simulink model "aracer"  (R2024b)
settings: Solver=FixedStepAuto  StartTime=0.0  StopTime=10.0  RelTol=1e-3
libraries: robotlib x4, simulink x2
settings Model: Creator=mrudi  LastModifiedBy=mrudi
settings OptimizationCC: DefaultParameterBehavior=Inlined  EnhancedBackFolding=on  PassReuseOutputArgsAs=Individual arguments  ZeroExternalMemoryAtStartup=off  ZeroInternalMemoryAtStartup=off  MaxStackSize=64  OptimizeBlockOrder=speed  DifferentSizesBufferReuse=on  OptimizationCustomize=off  EfficientTunableParamExpr=on
settings DebuggingCC: ParameterTunabilityLossMsg=error
settings HardwareCC: ProdBitPerPointer=32  ProdBitPerSizeT=32  ProdBitPerPtrDiffT=32  ProdLargestAtomicFloat=None  ProdIntDivRoundTo=Undefined  ProdEndianess=Unspecified  ProdWordSize=32  ProdHWDeviceType=Generic->Unspecified (assume 32-bit Generic)  UseEmbeddedCoderFeatures=off
settings SFSimCC: MATLABDynamicMemAlloc=off
settings RTWCC: Description=Embedded Coder  SystemTargetFile=ert.tlc  HardwareBoard=Robot Operating System (ROS)  TLCOptions="-aInlineSetEventsForThisBaseRateFcn=TLC_FALSE -aSuppressMultiTaskScheduler=TLC_FALSE  -aRateBasedStepFcn=0"  GenCodeOnly=on  TemplateMakefile=ert_default_tmf  Toolchain=Catkin  TargetLang=C++
settings CodeAppCC: ForceParamTrailComments=on  IgnoreCustomStorageClasses=off  OperatorAnnotations=on  SimulinkDataObjDesc=on  SFDataObjDesc=on  InsertBlockDesc=on
settings ERTTargetCC: SupportNonInlinedSFcns=on

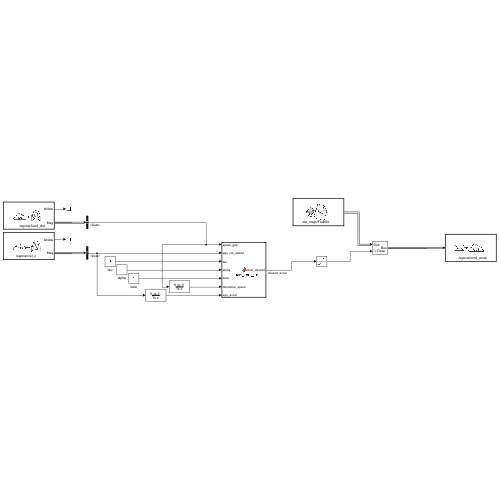
[thumbnail: Simulink's stored preview of the top-level diagram]
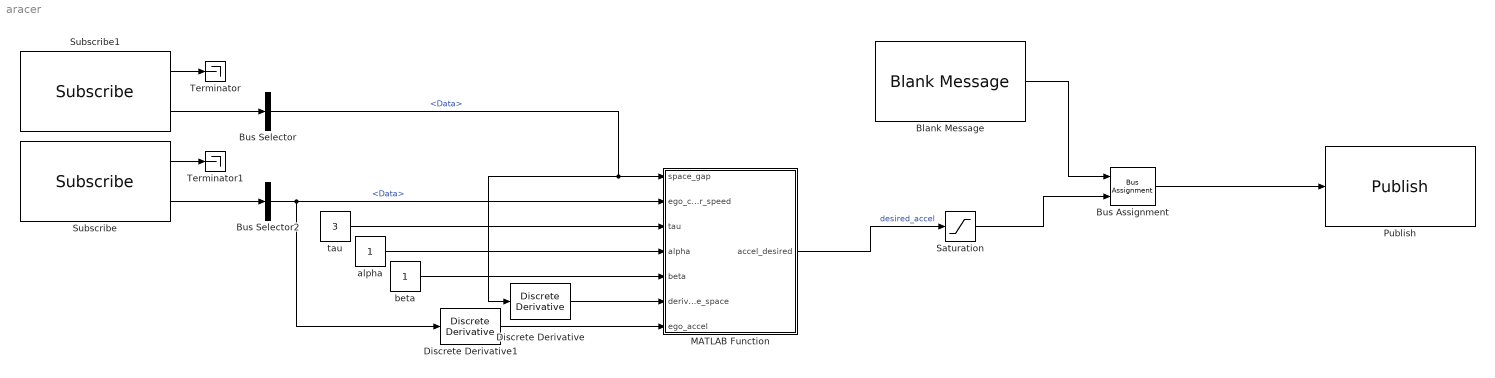
== system aracer ==
  Blank Message : robotlib/Blank Message  messageClass=Message  entityType=std_msgs/Float64  messageType=std_msgs/Float64  SampleTime=inf  legacyBusStruct=off
  Bus Assignment : BusAssignment  AssignedSignals=Data
  Bus Selector : BusSelector  OutputSignals=Data
  Bus Selector2 : BusSelector  OutputSignals=Data
  Discrete Derivative : simulink/Discrete/Discrete Derivative  gainval=1.0  ICPrevScaledInput=0.0  OutMin=[]  OutMax=[]  OutDataType=fixdt(1, 16)  OutScaling=2^-10  DoSatur=off
  Discrete Derivative1 : simulink/Discrete/Discrete Derivative  gainval=1.0  ICPrevScaledInput=0.0  OutMin=[]  OutMax=[]  OutDataType=fixdt(1, 16)  OutScaling=2^-10  DoSatur=off
  MATLAB Function : MATLAB Function  TreatAsAtomicUnit=on
  Publish : robotlib/Publish  topicSource=Specify your own  topic=/egocar/cmd_accel  messageType=std_msgs/Float64  legacyBusStruct=off  messageQueueLength=1
  Saturation : Saturate  UpperLimit=1.5  LowerLimit=-3.0
  Subscribe : robotlib/Subscribe  topicSource=Specify your own  topic=/egocar/vel_x  messageType=std_msgs/Float64  SampleTime=-1  legacyBusStruct=off  messageQueueLength=1
  Subscribe1 : robotlib/Subscribe  topicSource=Specify your own  topic=/egocar/lead_dist  messageType=std_msgs/Float64  SampleTime=-1  legacyBusStruct=off  messageQueueLength=1
  Terminator : Terminator
  Terminator1 : Terminator
  alpha : Constant
  beta : Constant
  tau : Constant  Value=3
  wires:
  Bus Assignment/1 -> Publish/1
  Subscribe1/1 -> Terminator/1
  Blank Message/1 -> Bus Assignment/1
  tau/1 -> MATLAB Function/3(tau)
  Subscribe/1 -> Terminator1/1
  Bus Selector2/1 -> MATLAB Function/2(ego_car_speed), Discrete Derivative1/1  "<Data>"
  alpha/1 -> MATLAB Function/4(alpha)
  Bus Selector/1 -> Discrete Derivative/1, MATLAB Function/1(space_gap)  "<Data>"
  Subscribe/2 -> Bus Selector2/1
  Subscribe1/2 -> Bus Selector/1
  Discrete Derivative/1 -> MATLAB Function/6(derivative_space)
  Discrete Derivative1/1 -> MATLAB Function/7(ego_accel)
  beta/1 -> MATLAB Function/5(beta)
  MATLAB Function/1(accel_desired) -> Saturation/1  "desired_accel"
  Saturation/1 -> Bus Assignment/2

== matlab function aracer/MATLAB Function ==
  data: space_gap input; accel_desired output; ego_car_speed input; tau input; alpha input; beta input; derivative_space input; ego_accel input
function accel_desired = constant_time_gap(space_gap, ego_car_speed, tau, alpha, beta, derivative_space, ego_accel)

accel_desired = alpha * (space_gap - tau * ego_car_speed) + beta * (derivative_space - tau * ego_accel);
